simulink library "eps_model_lib_2018b"  (R2018b)
settings: Solver=VariableStepAuto  StartTime=0.0  StopTime=10.0  RelTol=1e-3
undefined symbols (not defined in the file or in its folder): simParams
libraries: simulink x3, aerolibutil x1, solar_panels_lib x1
settings Model: Creator=Taylor  LastModifiedBy=Nick's PC

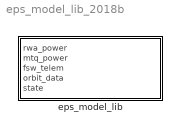
== system eps_model_lib_2018b ==
  eps_model_lib : Subsystem

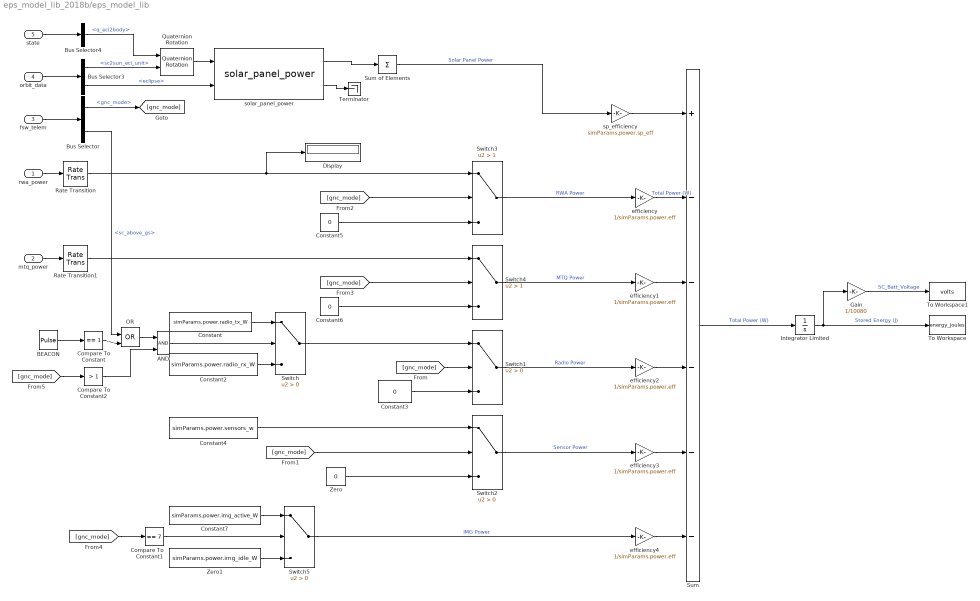
== system eps_model_lib_2018b/eps_model_lib ==
  rwa_power : Inport
  mtq_power : Inport  Port=2
  fsw_telem : Inport  Port=3  OutDataTypeStr=Bus: fsw_telemetry
  orbit_data : Inport  Port=4  OutDataTypeStr=Bus: orbit_data
  state : Inport  Port=5  OutDataTypeStr=Bus: state
  AND : Logic  IconShape=distinctive  AllPortsSameDT=off  OutDataTypeStr=boolean
  BEACON : DiscretePulseGenerator  PulseType=Time based  Period=60  PulseWidth=100 * (1.0 / 60)
  Bus Selector : BusSelector  OutputSignals=gnc_mode,sc_above_gs
  Bus Selector3 : BusSelector  OutputSignals=sc2sun_eci_unit,eclipse
  Bus Selector4 : BusSelector  OutputSignals=q_eci2body
  Compare To Constant : simulink/Logic and Bit Operations/Compare To Constant  relop===  const=1  OutDataTypeStr=boolean
  Compare To Constant1 : simulink/Logic and Bit Operations/Compare To Constant  relop===  const=7  OutDataTypeStr=boolean
  Compare To Constant2 : simulink/Logic and Bit Operations/Compare To Constant  relop=>  const=1  OutDataTypeStr=boolean
  Constant : Constant  Value=simParams.power.radio_tx_W
  Constant2 : Constant  Value=simParams.power.radio_rx_W
  Constant3 : Constant  Value=0
  Constant4 : Constant  Value=simParams.power.sensors_w
  Constant5 : Constant  Value=0
  Constant6 : Constant  Value=0
  Constant7 : Constant  Value=simParams.power.img_active_W
  Display : Display
  Gain : Gain  Gain=1/10080
  Integrator Limited : Integrator  InitialCondition=simParams.power.init_dod*simParams.power.batt_capacity  LimitOutput=on  UpperSaturationLimit=simParams.power.batt_capacity  LowerSaturationLimit=0
  OR : Logic  Operator=OR  IconShape=distinctive  AllPortsSameDT=off  OutDataTypeStr=boolean
  Quaternion Rotation : aerolibutil/Quaternion Rotation
  Rate Transition : RateTransition  OutPortSampleTime=simParams.sample_time_s
  Rate Transition1 : RateTransition  OutPortSampleTime=simParams.sample_time_s
  Sum : Sum  Inputs=+-----
  Sum of Elements : Sum  Inputs=+
  Switch{,1..2,5} (4 alike) : Switch  Criteria=u2 > Threshold
  Switch3 : Switch  Criteria=u2 > Threshold  Threshold=1
  Switch4 : Switch  Criteria=u2 > Threshold  Threshold=1
  Terminator : Terminator
  To Workspace : ToWorkspace  VariableName=energy_joules  SaveFormat=Timeseries  SampleTime=-1
  To Workspace1 : ToWorkspace  VariableName=volts  SaveFormat=Timeseries  SampleTime=-1
  Zero : Constant  Value=0  OutDataTypeStr=Inherit: Inherit via back propagation
  Zero1 : Constant  Value=simParams.power.img_idle_W  OutDataTypeStr=Inherit: Inherit via back propagation
  efficiency{,1..4} (5 alike) : Gain  Gain=1/simParams.power.eff
  solar_panel_power : solar_panels_lib/solar_panels_lib/solar_panel_power  SystemSampleTime=-1
  sp_efficiency : Gain  Gain=simParams.power.sp_eff
  wires:
  Switch4/1 -> efficiency1/1  "MTQ Power"
  Sum/1 -> Integrator Limited/1  "Total Power (W)"
  Bus Selector3/1 -> Quaternion Rotation/2  "<sc2sun_eci_unit>"
  Sum of Elements/1 -> sp_efficiency/1  "Solar Panel Power"
  solar_panel_power/1 -> Sum of Elements/1
  solar_panel_power/2 -> Terminator/1
  Quaternion Rotation/1 -> solar_panel_power/1
  Bus Selector4/1 -> Quaternion Rotation/1  "<q_eci2body>"
  Bus Selector/2 -> OR/1  "<sc_above_gs>"
  BEACON/1 -> Compare To Constant/1
  OR/1 -> AND/1
  Constant/1 -> Switch/1
  Constant2/1 -> Switch/3
  Constant3/1 -> Switch1/3
  Switch/1 -> Switch1/1
  Bus Selector/1 -> [gnc_mode]  "<gnc_mode>"
  [gnc_mode] -> Switch1/2
  Switch1/1 -> efficiency2/1  "Radio Power"
  [gnc_mode] -> Switch2/2
  Zero/1 -> Switch2/3
  Switch2/1 -> efficiency3/1  "Sensor Power"
  Constant4/1 -> Switch2/1
  [gnc_mode] -> Switch3/2
  Constant5/1 -> Switch3/3
  Constant6/1 -> Switch4/3
  [gnc_mode] -> Switch4/2
  [gnc_mode] -> Compare To Constant1/1
  Compare To Constant1/1 -> Switch5/2
  Integrator Limited/1 -> Gain/1, To Workspace/1  "Stored Energy (J)"
  Constant7/1 -> Switch5/1
  Zero1/1 -> Switch5/3
  Switch5/1 -> efficiency4/1  "IMG Power"
  Switch3/1 -> efficiency/1  "RWA Power"
  state/1 -> Bus Selector4/1
  orbit_data/1 -> Bus Selector3/1
  fsw_telem/1 -> Bus Selector/1
  rwa_power/1 -> Rate Transition/1
  mtq_power/1 -> Rate Transition1/1
  AND/1 -> Switch/2
  [gnc_mode] -> Compare To Constant2/1
  Compare To Constant2/1 -> AND/2
  Rate Transition/1 -> Display/1, Switch3/1
  Rate Transition1/1 -> Switch4/1
  sp_efficiency/1 -> Sum/1
  efficiency/1 -> Sum/2  "Total Power (W)"
  efficiency1/1 -> Sum/3
  efficiency2/1 -> Sum/4
  efficiency3/1 -> Sum/5
  efficiency4/1 -> Sum/6
  Compare To Constant/1 -> OR/2
  Gain/1 -> To Workspace1/1  "SC_Batt_Voltage"
  Bus Selector3/2 -> solar_panel_power/2  "<eclipse>"
